simulink model "hdl_generation"  (R2024b)
settings: Solver=VariableStepAuto  StartTime=0.0  StopTime=0.01  RelTol=1e-3
libraries: slpidlib x2, matrix_library x1, aerolibutil x1
settings Model: Creator=keybo  LastModifiedBy=keybo
settings OptimizationCC: BlockReduction=off  ConditionallyExecuteInputs=off  DefaultParameterBehavior=Inlined  UseFloatMulNetSlope=on
settings DebuggingCC: AlgebraicLoopMsg=error  MultiTaskCondExecSysMsg=warning  MultiTaskRateTransMsg=warning  SingleTaskRateTransMsg=warning  FrameProcessingCompatibilityMsg=warning  NonCurrentReleaseOperatingPointMsg=warning
settings HardwareCC: ProdBitPerPointer=32  ProdBitPerSizeT=32  ProdBitPerPtrDiffT=32  ProdLargestAtomicFloat=None  ProdIntDivRoundTo=Undefined  ProdEndianess=Unspecified  ProdWordSize=32  ProdHWDeviceType=ASIC/FPGA->ASIC/FPGA  TargetBitPerLong=64  TargetBitPerPointer=64  TargetBitPerSizeT=64  TargetBitPerPtrDiffT=64  TargetLongLongMode=on  TargetIntDivRoundTo=Zero  TargetEndianess=LittleEndian  TargetWordSize=64  TargetHWDeviceType=Custom Processor->MATLAB Host Computer  ProdEqTarget=off

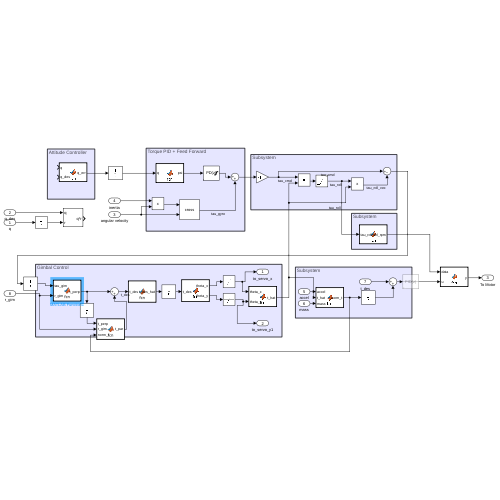
[thumbnail: Simulink's stored preview of the top-level diagram]
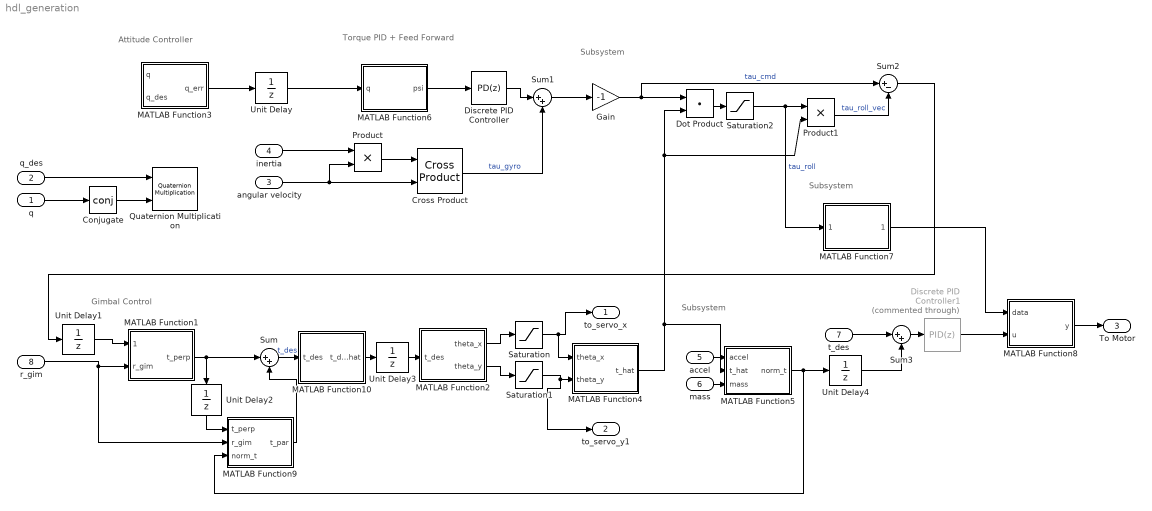
== system hdl_generation ==
  note: Subsystem
  note: Subsystem
  note: Torque PID + Feed Forward
  note: Subsystem
  note: Attitude Controller
  note: Gimbal Control
  q : Inport  PortDimensions=4
  q_des : Inport  Port=2  PortDimensions=4
  angular velocity : Inport  Port=3  PortDimensions=3
  inertia : Inport  Port=4
  accel : Inport  Port=5  PortDimensions=3
  mass : Inport  Port=6  PortDimensions=1
  t_des : Inport  Port=7  PortDimensions=3
  r_gim : Inport  Port=8  PortDimensions=3
  Conjugate : Math  Operator=conj  SignedPower=on  RndMeth=Zero
  Cross Product : matrix_library/Cross Product
  Discrete PID Controller : slpidlib/PID Controller  Controller=PD  Form=Parallel  TimeDomain=Discrete-time  UseExternalTs=off  SampleTime=0.001  IntegratorMethod=Forward Euler  FilterMethod=Forward Euler  ControllerParametersSource=internal  P=1  I=1  UseKiTs=off  D=1  UseExternalDerivativeSource=off  N=1  UseFilter=on  TunerSelectOption=Transfer Function Based (PID Tuner App)  InitialConditionSource=internal  InitialConditionForIntegrator=0  InitialConditionForFilter=1  DifferentiatorICPrevScaledInput=0  ExternalReset=none  TrackingMode=off  Kt=1  LimitOutput=on  SatLimitsSource=internal  UpperSaturationLimit=10  LowerSaturationLimit=-10  LinearizeAsGain=off  AntiWindupMode=none  Kb=1  LimitIntegrator=off  UpperIntegratorSaturationLimit=inf  LowerIntegratorSaturationLimit=-inf  POutMin=[]  POutMax=[]  IOutMin=[]  IOutMax=[]  DOutMin=[]  DOutMax=[]  NOutMin=[]  NOutMax=[]  SumOutMin=[]  SumOutMax=[]  SaturationOutMin=[]  SaturationOutMax=[]  PParamMin=[]  PParamMax=[]  IParamMin=[]  IParamMax=[]  DParamMin=[]  DParamMax=[]  NParamMin=[]  NParamMax=[]  KbParamMin=[]  KbParamMax=[]  KtParamMin=[]  KtParamMax=[]  KbOutMin=[]  KbOutMax=[]  KtOutMin=[]  KtOutMax=[]  IntegratorOutMin=[]  IntegratorOutMax=[]  FilterOutMin=[]  FilterOutMax=[]  SumI1OutMin=[]  SumI1OutMax=[]  SumI2OutMin=[]  SumI2OutMax=[]  SumI3OutMin=[]  SumI3OutMax=[]  SumI4OutMin=[]  SumI4OutMax=[]  SumDOutMin=[]  SumDOutMax=[]  DifferentiatorOutMin=[]  DifferentiatorOutMax=[]  FilterDiffOutCoefMin=[]  FilterDiffOutCoefMax=[]  ReciprocalOutMin=[]  ReciprocalOutMax=[]  SumDenOutMin=[]  SumDenOutMax=[]  SumNumOutMin=[]  SumNumOutMax=[]  DivideOutMin=[]  DivideOutMax=[]  UdiffTsProdOutMin=[]  UdiffTsProdOutMax=[]  NTsProdOutMin=[]  NTsProdOutMax=[]  UintegralTsProdOutMin=[]  UintegralTsProdOutMax=[]  UngainTsProdOutMin=[]  UngainTsProdOutMax=[]  ClampingZeroOutDataTypeStr=Inherit: Inherit via back propagation  ClampingZeroOutMin=[]  ClampingZeroOutMax=[]  FilterDenConstantOutDataTypeStr=Inherit: Inherit via back propagation  FilterDenConstantOutMin=[]  FilterDenConstantOutMax=[]  PCopyOutDataTypeStr=Inherit: Inherit via back propagation  PCopyOutMin=[]  PCopyOutMax=[]  NCopyOutDataTypeStr=Inherit: Inherit via back propagation  NCopyOutMin=[]  NCopyOutMax=[]  IntegratorContinuousStateAttributes=''  IntegratorStateMustResolveToSignalObject=off  IntegratorRTWStateStorageClass=Auto  FilterContinuousStateAttributes=''  FilterStateMustResolveToSignalObject=off  FilterRTWStateStorageClass=Auto  ParallelPVariant=InternalParameters  IdealPVariant=Disabled  IVariant=Disabled  DVariant=InternalParameters  IntegratorVariant=Disabled  SatVariant=Enabled  AWVariant=Disabled  PCopyVariant=Disabled  TRVariant=Disabled  FdbkBlocksVariant=Forward  IdealPFdbkVariant=Disabled  SatFdbkVariant=Disabled  DerivativeFilterVariant=ForwardEulerFilter  NVariant=InternalParameters  NCopyVariant=Disabled  FilterICVariant=InternalICsFilter  IntegratorICVariant=Disabled  ExternalResetVariant=Disabled  TRSumVariant=Passthrough  SumFdbkVariant=Disabled  SumVariant=Sum_PD  TsampFilterVariant=InternalTs  TsampNgainVariant=Passthrough  TsampIntegralVariant=Disabled_SignalSpec  ExternalSaturationOutDataTypeStr=Inherit: Same as second input  DerivativeSourceVariant=ErrorSignal  PreIntVariant=InternalPreInt
      settings: LibrarySourceBlock=hdlsllib/Discrete/Discrete PID Controller
  Discrete PID Controller1 : slpidlib/PID Controller  Commented=through  Controller=PID  Form=Parallel  TimeDomain=Discrete-time  UseExternalTs=off  SampleTime=0.001  IntegratorMethod=Forward Euler  FilterMethod=Forward Euler  ControllerParametersSource=internal  P=0  I=1  UseKiTs=off  D=1  UseExternalDerivativeSource=off  N=100  UseFilter=on  TunerSelectOption=Transfer Function Based (PID Tuner App)  InitialConditionSource=internal  InitialConditionForIntegrator=0  InitialConditionForFilter=0  DifferentiatorICPrevScaledInput=0  ExternalReset=none  TrackingMode=off  Kt=1  LimitOutput=off  SatLimitsSource=internal  UpperSaturationLimit=inf  LowerSaturationLimit=-inf  LinearizeAsGain=off  AntiWindupMode=none  Kb=1  LimitIntegrator=off  UpperIntegratorSaturationLimit=inf  LowerIntegratorSaturationLimit=-inf  POutMin=[]  POutMax=[]  IOutMin=[]  IOutMax=[]  DOutMin=[]  DOutMax=[]  NOutMin=[]  NOutMax=[]  SumOutMin=[]  SumOutMax=[]  SaturationOutMin=[]  SaturationOutMax=[]  PParamMin=[]  PParamMax=[]  IParamMin=[]  IParamMax=[]  DParamMin=[]  DParamMax=[]  NParamMin=[]  NParamMax=[]  KbParamMin=[]  KbParamMax=[]  KtParamMin=[]  KtParamMax=[]  KbOutMin=[]  KbOutMax=[]  KtOutMin=[]  KtOutMax=[]  IntegratorOutMin=[]  IntegratorOutMax=[]  FilterOutMin=[]  FilterOutMax=[]  SumI1OutMin=[]  SumI1OutMax=[]  SumI2OutMin=[]  SumI2OutMax=[]  SumI3OutMin=[]  SumI3OutMax=[]  SumI4OutMin=[]  SumI4OutMax=[]  SumDOutMin=[]  SumDOutMax=[]  DifferentiatorOutMin=[]  DifferentiatorOutMax=[]  FilterDiffOutCoefMin=[]  FilterDiffOutCoefMax=[]  ReciprocalOutMin=[]  ReciprocalOutMax=[]  SumDenOutMin=[]  SumDenOutMax=[]  SumNumOutMin=[]  SumNumOutMax=[]  DivideOutMin=[]  DivideOutMax=[]  UdiffTsProdOutMin=[]  UdiffTsProdOutMax=[]  NTsProdOutMin=[]  NTsProdOutMax=[]  UintegralTsProdOutMin=[]  UintegralTsProdOutMax=[]  UngainTsProdOutMin=[]  UngainTsProdOutMax=[]  ClampingZeroOutDataTypeStr=Inherit: Inherit via back propagation  ClampingZeroOutMin=[]  ClampingZeroOutMax=[]  FilterDenConstantOutDataTypeStr=Inherit: Inherit via back propagation  FilterDenConstantOutMin=[]  FilterDenConstantOutMax=[]  PCopyOutDataTypeStr=Inherit: Inherit via back propagation  PCopyOutMin=[]  PCopyOutMax=[]  NCopyOutDataTypeStr=Inherit: Inherit via back propagation  NCopyOutMin=[]  NCopyOutMax=[]  IntegratorContinuousStateAttributes=''  IntegratorStateMustResolveToSignalObject=off  IntegratorRTWStateStorageClass=Auto  FilterContinuousStateAttributes=''  FilterStateMustResolveToSignalObject=off  FilterRTWStateStorageClass=Auto  ParallelPVariant=InternalParameters  IdealPVariant=Disabled  IVariant=InternalParameters  DVariant=InternalParameters  IntegratorVariant=Discrete  SatVariant=Disabled  AWVariant=Passthrough  PCopyVariant=Disabled  TRVariant=Disabled  FdbkBlocksVariant=Forward  IdealPFdbkVariant=Disabled  SatFdbkVariant=Disabled  DerivativeFilterVariant=ForwardEulerFilter  NVariant=InternalParameters  NCopyVariant=Disabled  FilterICVariant=InternalICsFilter  IntegratorICVariant=InternalICs  ExternalResetVariant=Disabled  TRSumVariant=Passthrough  SumFdbkVariant=Disabled  SumVariant=Sum_PID  TsampFilterVariant=InternalTs  TsampNgainVariant=Passthrough  TsampIntegralVariant=Disabled_SignalSpec  ExternalSaturationOutDataTypeStr=Inherit: Same as second input  DerivativeSourceVariant=ErrorSignal  PreIntVariant=InternalPreInt
      settings: LibrarySourceBlock=simulink/Discrete/Discrete PID Controller
  Dot Product : DotProduct  OutDataTypeStr=Inherit: Inherit via internal rule
  Gain : Gain  Gain=-1
  MATLAB Function1 : MATLAB Function  TreatAsAtomicUnit=on
  MATLAB Function10 : MATLAB Function  TreatAsAtomicUnit=on
  MATLAB Function2 : MATLAB Function  TreatAsAtomicUnit=on
  MATLAB Function3 : MATLAB Function  TreatAsAtomicUnit=on
  MATLAB Function4 : MATLAB Function  TreatAsAtomicUnit=on
  MATLAB Function5 : MATLAB Function  TreatAsAtomicUnit=on
  MATLAB Function6 : MATLAB Function  TreatAsAtomicUnit=on
  MATLAB Function7 : MATLAB Function  TreatAsAtomicUnit=on
  MATLAB Function8 : MATLAB Function  TreatAsAtomicUnit=on
  MATLAB Function9 : MATLAB Function  TreatAsAtomicUnit=on
  Product : Product
  Product1 : Product
  Quaternion Multiplication : aerolibutil/Quaternion Multiplication
  Saturation : Saturate
  Saturation1 : Saturate
  Saturation2 : Saturate
  Sum : Sum  Inputs=|++
  Sum1 : Sum  Inputs=|++
  Sum2 : Sum  Inputs=|+-
  Sum3 : Sum  Inputs=|++
  Unit Delay{,1..3} (4 alike) : UnitDelay  SampleTime=-1  HasFrameUpgradeWarning=on
  Unit Delay4 : UnitDelay  SampleTime=0.001  HasFrameUpgradeWarning=on
  to_servo_x : Outport  PortDimensions=1
  to_servo_y1 : Outport  Port=2  PortDimensions=1
  To Motor : Outport  Port=3
  wires:
  MATLAB Function10/1(t_des_hat) -> Unit Delay3/1
  MATLAB Function2/1(theta_x) -> Saturation/1
  Saturation/1 -> to_servo_x/1, MATLAB Function4/1(theta_x)
  Product/1 -> Cross Product/1
  Saturation1/1 -> to_servo_y1/1, MATLAB Function4/2(theta_y)
  q_des/1 -> Quaternion Multiplication/1
  inertia/1 -> Product/1
  r_gim/1 -> MATLAB Function1/2(r_gim), MATLAB Function9/2(r_gim)
  MATLAB Function6/1(psi) -> Discrete PID Controller/1
  Discrete PID Controller/1 -> Sum1/1
  MATLAB Function2/2(theta_y) -> Saturation1/1
  Cross Product/1 -> Sum1/2  "tau_gyro"
  MATLAB Function5/1(norm_t) -> Unit Delay4/1, MATLAB Function9/3(norm_t)
  angular velocity/1 -> Cross Product/2, Product/2
  MATLAB Function3/1(q_err) -> Unit Delay/1
  Sum/1 -> MATLAB Function10/1(t_des)  "t_des"
  MATLAB Function9/1(t_par) -> Sum/2
  q/1 -> Conjugate/1
  accel/1 -> MATLAB Function5/1(accel)
  t_des/1 -> Sum3/1
  mass/1 -> MATLAB Function5/3(mass)
  MATLAB Function8/1(y) -> To Motor/1
  Discrete PID Controller1/1 -> MATLAB Function8/2(u)
  MATLAB Function7/1(del_rpm) -> MATLAB Function8/1(data)
  Sum2/1 -> Unit Delay1/1
  MATLAB Function4/1(t_hat) -> MATLAB Function5/2(t_hat), Product1/2, Dot Product/2
  Saturation2/1 -> MATLAB Function7/1(tau_roll), Product1/1  "tau_roll"
  Gain/1 -> Sum2/1, Dot Product/1  "tau_cmd"
  Sum1/1 -> Gain/1
  Product1/1 -> Sum2/2  "tau_roll_vec"
  Dot Product/1 -> Saturation2/1
  Unit Delay/1 -> MATLAB Function6/1(q)
  Unit Delay1/1 -> MATLAB Function1/1(tau_gim)
  MATLAB Function1/1(t_perp) -> Sum/1, Unit Delay2/1
  Unit Delay2/1 -> MATLAB Function9/1(t_perp)
  Unit Delay3/1 -> MATLAB Function2/1(t_des)
  Sum3/1 -> Discrete PID Controller1/1
  Unit Delay4/1 -> Sum3/2
  Conjugate/1 -> Quaternion Multiplication/2

== matlab function hdl_generation/MATLAB Function1 ==
  data: tau_gim input; t_perp output; r_gim input
function t_perp = fcn(tau_gim, r_gim)

    %t_perp = (cross(tau_gim, r_gim))/(norm(r_gim)^2); 
t_perp = tau_gim+r_gim;

== matlab function hdl_generation/MATLAB Function10 ==
  data: t_des input; t_des_hat output
function t_des_hat = fcn(t_des)
t_des_hat = t_des;
%t_des_hat = t_des/norm(t_des);

== matlab function hdl_generation/MATLAB Function4 ==
  data: theta_x input; t_hat output; theta_y input
function t_hat  = fcn(theta_x, theta_y)

%t_hat = [sin(theta_y)
%    -sin(theta_x)*cos(theta_y)
%    cos(theta_x)*cos(theta_y)];

t_hat = [1
    -1
    1];

== matlab function hdl_generation/MATLAB Function9 ==
  data: t_perp input; t_par output; r_gim input; norm_t input
function t_par = fcn(t_perp, r_gim, norm_t)

%t_par = sqrt(norm_t^2 - norm(t_perp)^2)*r_gim/norm(r_gim);   
t_par = t_perp+r_gim+norm_t;

== matlab function hdl_generation/MATLAB Function6 ==
  data: q input; psi output
function psi  = fcn(q)

q_0 = q(1);
v = [q(2)
    q(3)
    q(4)];
psi_comp = 2*atan2(norm(v), q_0)*v/norm(v);
%psi_comp = q_0*v;
psi = sign(psi_comp).*psi_comp;

== matlab function hdl_generation/MATLAB Function8 ==
  data: data input; y output; u input
function y = fcn(data, u)

y = u;

== matlab function hdl_generation/MATLAB Function7 ==
  data: tau_roll input; del_rpm output
function del_rpm = fcn(tau_roll)

del_rpm = tau_roll;

== matlab function hdl_generation/MATLAB Function5 ==
  data: accel input; norm_t output; t_hat input; mass input
function norm_t = fcn(accel, t_hat, mass)

%norm_t = mass*(dot(accel, t_hat));
norm_t = mass*t_hat;

== matlab function hdl_generation/MATLAB Function2 ==
  data: t_des input; theta_x output; theta_y output
function [theta_x, theta_y] = fcn(t_des)

%theta_x = -atan2(t_des(2), t_des(3)); % t_des(2) and (3) are y and z axes
%theta_y = asin(t_des(1)); % t_des(1) is on x axis 
theta_x = 1;
theta_y = 1;

== matlab function hdl_generation/MATLAB Function3 ==
  data: q input; q_err output; q_des input
function q_err = fcn(q, q_des)

q = q.';
q_des = q_des.';
%q_err = quatmultiply(q_des, conj(q));

q_err = q;
